simulink model "gtm_design_baseline3"  (R2023b)
settings: Solver=ode3  StartTime=0.0  StopTime=15  FixedStep=Timestep  MaxStep=.1  RelTol=1e-5
StopFcn:
  | MWSout=grabmws(bdroot);
  | MWSout.lastrun=datestr(now);
values from neighbouring files (symbols this model uses):
  f0_att = fc_att*Kb_att/Kb_rate    (= 0.125)    [runmain.m]    (also in runmain_match.m = 0.05)
  fc_att = 1/2    (= 0.5)    [runmain.m]    (also in runmain_match.m)
  fc_rate = 1/2    (= 0.5)    [runmain.m]    (also in runmain_match.m = 0)
  fi_att = 1/4    (= 0.25)    [runmain.m]    (also in runmain_match.m)
  fi_rate = 1/4    (= 0.25)    [runmain.m]    (also in runmain_match.m)
  flag_cmd = 0    [runmain.m]    (also in runmain_match.m)
  invBmat = inv(Bmat)    [runmain.m]    (also in runmain_match.m)
  invJ = inv(J)    [runmain.m]    (also in runmain_match.m)
  J = [Ixx 0 -Ixz; 0 Iyy 0; -Ixz 0 Izz]    [runmain.m]    (also in runmain_match.m)
  Kb_att = 1    [runmain.m]    (also in runmain_match.m)
  Kb_rate = 4    [runmain.m]    (also in runmain_match.m = 10)
  mws_designpoint = trimgtm(struct('eas',75,'gamma',0),'elev',1)    [runmain.m]    (also in runmain_match.m = trimgtm(struct('eas',90,'gamma',0),'elev',1))
undefined symbols (not defined in the file or in its folder): Aero, aftfuel, aftfuel_pos, b, bias, Cbar, cg_pos0, cg_shift_gear, DamageCase, DamageModels, DamageOnsetTime, engl_ang, engl_pos, engr_ang, engr_pos, fwdfuel, fwdfuel_pos, Inertia0, Inertia_shift_gear, ref_cg, runway_alt, S, StatesInp, symmetric_aero_on, Timestep, w0, WindDir, WindSpd
libraries: simulink_need_slupdate x56, Servo_Model_lib x18, Cross_Product_3D_lib x5, simulink x5, GTM_aerolib x4, Polyval_lib x3, Euler_to_DCM_lib x2, eomlib x2, Vb_Converter_lib x1, sensors_T2_design_lib x1, Doublet_Generator_lib x1, NamedStore_lib x1
(part 2 of 4)

== system gtm_design_baseline3/Aircraft Model/EOM/State Labels ==
  I : Inport
  Bus Creator : BusCreator  Inputs=12
  Demux : Demux  Outputs=12
      settings: DisplayOption=none
  O : Outport  VectorParamsAs1DForOutWhenUnconnected=off
  wires:
  Demux/12 -> Bus Creator/12  "psi"
  Demux/9 -> Bus Creator/9  "altitude"
  Demux/8 -> Bus Creator/8  "longitude"
  Demux/7 -> Bus Creator/7  "latitude"
  Demux/6 -> Bus Creator/6  "rb"
  Demux/5 -> Bus Creator/5  "qb"
  Demux/4 -> Bus Creator/4  "pb"
  Demux/3 -> Bus Creator/3  "wb"
  Demux/2 -> Bus Creator/2  "vb"
  Demux/1 -> Bus Creator/1  "ub"
  I/1 -> Demux/1
  Demux/10 -> Bus Creator/10  "phi"
  Demux/11 -> Bus Creator/11  "theta"
  Bus Creator/1 -> O/1

== system gtm_design_baseline3/Aircraft Model/EOM/Xdot Labels ==
  I : Inport
  Bus Creator : BusCreator  Inputs=12
  Demux : Demux  Outputs=12
      settings: DisplayOption=none
  O : Outport  VectorParamsAs1DForOutWhenUnconnected=off
  wires:
  Bus Creator/1 -> O/1
  Demux/11 -> Bus Creator/11  "theta_dot"
  Demux/10 -> Bus Creator/10  "phi_dot"
  I/1 -> Demux/1
  Demux/1 -> Bus Creator/1  "ub_dot"
  Demux/2 -> Bus Creator/2  "vb_dot"
  Demux/3 -> Bus Creator/3  "wb_dot"
  Demux/4 -> Bus Creator/4  "pb_dot"
  Demux/5 -> Bus Creator/5  "qb_dot"
  Demux/6 -> Bus Creator/6  "rb_dot"
  Demux/7 -> Bus Creator/7  "latitude_dot"
  Demux/8 -> Bus Creator/8  "longitude_dot"
  Demux/9 -> Bus Creator/9  "altitude_dot"
  Demux/12 -> Bus Creator/12  "psi_dot"

== system gtm_design_baseline3/Aircraft Model/Engines/3D Vector Cross Product ==
  A : Inport
  B : Inport  Port=2
  Demux : Demux  Outputs=3
      settings: DisplayOption=none
  Demux1 : Demux  Outputs=3
      settings: DisplayOption=none
  Gain : Gain  Gain=-1  SaturateOnIntegerOverflow=on  OutDataTypeStr=Inherit: Same as input  ParamDataTypeStr=Inherit: Same as input
  Ground : Ground
  Mux : Mux  Inputs=9
  Product : Product  Multiplication=Matrix(*)  SaturateOnIntegerOverflow=on  OutDataTypeStr=Inherit: Same as first input
  Reshape : Reshape  OutputDimensionality=Customize  OutputDimensions=[3,3]
  AxB : Outport  VectorParamsAs1DForOutWhenUnconnected=off
  wires:
  B/1 -> Product/2
  Reshape/1 -> Product/1
  Mux/1 -> Reshape/1
  Demux1/1 -> Mux/8
  Demux/2 -> Mux/7
  Demux/1 -> Mux/6
  Demux1/3 -> Mux/4
  Demux1/2 -> Mux/3
  Demux/3 -> Mux/2
  Gain/1 -> Demux1/1
  Ground/1 -> Mux/9, Mux/5, Mux/1
  Product/1 -> AxB/1
  A/1 -> Gain/1, Demux/1

== system gtm_design_baseline3/Aircraft Model/Engines/CG torque ==
  AC : Inport
  Lthrust : Inport  Port=2
  Rthrust : Inport  Port=3
  3D Vector Cross Product : Cross_Product_3D_lib/3D Vector Cross Product  SystemSampleTime=-1  VariantActivationTime=update diagram  AllowFlexibleInterface=on  Latency=0  AutoFrameSizeCalculation=off
  3D Vector Cross Product1 : Cross_Product_3D_lib/3D Vector Cross Product  SystemSampleTime=-1  VariantActivationTime=update diagram  AllowFlexibleInterface=on  Latency=0  AutoFrameSizeCalculation=off
  Bus Selector30 : BusSelector  OutputSignals=LfEng,CG,RtEng
  Sum1 : Sum  InputSameDT=on  SaturateOnIntegerOverflow=on  OutDataTypeStr=Inherit: Same as first input
  Sum6 : Sum  Inputs=+-  InputSameDT=on  SaturateOnIntegerOverflow=on  OutDataTypeStr=Inherit: Same as first input
  Sum7 : Sum  Inputs=-+  InputSameDT=on  SaturateOnIntegerOverflow=on  OutDataTypeStr=Inherit: Same as first input
  Torques : Outport  VectorParamsAs1DForOutWhenUnconnected=off
  wires:
  AC/1 -> Bus Selector30/1
  Bus Selector30/2 -> Sum7/1, Sum6/2  "<CG>"
  Lthrust/1 -> 3D Vector Cross Product1/2
  Rthrust/1 -> 3D Vector Cross Product/2
  Sum7/1 -> 3D Vector Cross Product/1
  Sum6/1 -> 3D Vector Cross Product1/1
  3D Vector Cross Product1/1 -> Sum1/1
  3D Vector Cross Product/1 -> Sum1/2
  Sum1/1 -> Torques/1
  Bus Selector30/3 -> Sum7/2  "<RtEng>"
  Bus Selector30/1 -> Sum6/1  "<LfEng>"

== system gtm_design_baseline3/Aircraft Model/Engines/Jetcat P70 (Left) ==
  note: No longer "halved"
  Throttle : Inport
  pratio : Inport  Port=2
  tratio : Inport  Port=3
  BypassDynamics : Inport  Port=4
  Fuel Pump Voltage : Lookup  InputValues=fuelflow_table  Table=fuelpump_table  LookUpMeth=Interpolation-Use End Values  SaturateOnIntegerOverflow=off
  Product2 : Product  RndMeth=Zero
  RPMref_2_EGT : Polyval  Coefs=Coeff_EGT
  RPMref_2_FuelFlow : Polyval  Coefs=Coeff_fuelflow
  RPMref_2_Thrust : Polyval  Coefs=Coeff_thrust
  Sum : Sum  Inputs=|+-
  Switch : Switch  Criteria=u2 ~= 0  SaturateOnIntegerOverflow=off  InputSameDT=off
  Terminator : Terminator
  Throttle1 : InportShadow
  Throttle2 : InportShadow
  Throttle_2_RPMref : Polyval  Coefs=Coeff_throttle
  Tunable Lag : Subsystem
  UnScale_Ref_RPM : Gain  Gain=123000/100
  Variable Lag : MATLAB Function  TreatAsAtomicUnit=on
  angular momentum : Gain  Gain=(pi*shaft_dia^4/32) * shaft_len * density * (2*pi/60)
  Thrust (lbf) : Outport  VectorParamsAs1DForOutWhenUnconnected=off
  RPM : Outport  Port=2  VectorParamsAs1DForOutWhenUnconnected=off
  h (slg-ft^2/s) : Outport  Port=3  VectorParamsAs1DForOutWhenUnconnected=off
  Fuel Flow (lbs/min) : Outport  Port=4  VectorParamsAs1DForOutWhenUnconnected=off
  Fuel Pump Voltage (V) : Outport  Port=5  VectorParamsAs1DForOutWhenUnconnected=off
  EGT (deg C) : Outport  Port=6  VectorParamsAs1DForOutWhenUnconnected=off
  wires:
  Throttle2/1 -> Switch/1
  BypassDynamics/1 -> Switch/2
  Tunable Lag/1(y) -> Switch/3, Sum/2  "Throttle_Lag"
  Switch/1 -> Throttle_2_RPMref/1
  Variable Lag/1(tau) -> Tunable Lag/1(tau)  "tau"
  Throttle/1 -> Tunable Lag/2(throttle)
  Throttle_2_RPMref/1 -> RPMref_2_EGT/1, Variable Lag/1(pa), RPMref_2_Thrust/1, UnScale_Ref_RPM/1, RPMref_2_FuelFlow/1
  angular momentum/1 -> h (slg-ft^2/s)/1
  UnScale_Ref_RPM/1 -> angular momentum/1, RPM/1
  tratio/1 -> Terminator/1
  RPMref_2_Thrust/1 -> Product2/1
  Product2/1 -> Thrust (lbf)/1
  RPMref_2_FuelFlow/1 -> Fuel Flow (lbs/min)/1, Fuel Pump Voltage/1
  pratio/1 -> Product2/2
  Fuel Pump Voltage/1 -> Fuel Pump Voltage (V)/1
  RPMref_2_EGT/1 -> EGT (deg C)/1
  Sum/1 -> Variable Lag/2(dp)
  Throttle1/1 -> Sum/1

== system gtm_design_baseline3/Aircraft Model/Engines/Jetcat P70 (Right) ==
  note: No longer "halved"
  Throttle : Inport
  pratio : Inport  Port=2
  tratio : Inport  Port=3
  BypassDynamics : Inport  Port=4
  Fuel Pump Voltage : Lookup  InputValues=fuelflow_table  Table=fuelpump_table  LookUpMeth=Interpolation-Use End Values  SaturateOnIntegerOverflow=off
  Product2 : Product  RndMeth=Zero
  RPMref_2_EGT : Polyval  Coefs=Coeff_EGT
  RPMref_2_FuelFlow : Polyval  Coefs=Coeff_fuelflow
  RPMref_2_Thrust : Polyval  Coefs=Coeff_thrust
  Sum : Sum  Inputs=|+-
  Switch : Switch  Criteria=u2 ~= 0  SaturateOnIntegerOverflow=off  InputSameDT=off
  Terminator : Terminator
  Throttle1 : InportShadow
  Throttle2 : InportShadow
  Throttle_2_RPMref : Polyval  Coefs=Coeff_throttle
  Tunable Lag : Subsystem
  UnScale_Ref_RPM : Gain  Gain=123000/100
  Variable Lag : MATLAB Function  TreatAsAtomicUnit=on
  angular momentum : Gain  Gain=(pi*shaft_dia^4/32) * shaft_len * density * (2*pi/60)
  Thrust (lbf) : Outport  VectorParamsAs1DForOutWhenUnconnected=off
  RPM : Outport  Port=2  VectorParamsAs1DForOutWhenUnconnected=off
  h (slg-ft^2/s) : Outport  Port=3  VectorParamsAs1DForOutWhenUnconnected=off
  Fuel Flow (lbs/min) : Outport  Port=4  VectorParamsAs1DForOutWhenUnconnected=off
  Fuel Pump Voltage (V) : Outport  Port=5  VectorParamsAs1DForOutWhenUnconnected=off
  EGT (deg C) : Outport  Port=6  VectorParamsAs1DForOutWhenUnconnected=off
  wires:
  Throttle2/1 -> Switch/1
  BypassDynamics/1 -> Switch/2
  Tunable Lag/1(y) -> Switch/3, Sum/2  "Throttle_Lag"
  Switch/1 -> Throttle_2_RPMref/1
  Variable Lag/1(tau) -> Tunable Lag/1(tau)  "tau"
  Throttle/1 -> Tunable Lag/2(throttle)
  Throttle_2_RPMref/1 -> RPMref_2_FuelFlow/1, RPMref_2_EGT/1, RPMref_2_Thrust/1, UnScale_Ref_RPM/1, Variable Lag/1(pa)
  angular momentum/1 -> h (slg-ft^2/s)/1
  UnScale_Ref_RPM/1 -> angular momentum/1, RPM/1
  tratio/1 -> Terminator/1
  RPMref_2_Thrust/1 -> Product2/1
  Product2/1 -> Thrust (lbf)/1
  RPMref_2_FuelFlow/1 -> Fuel Flow (lbs/min)/1, Fuel Pump Voltage/1
  pratio/1 -> Product2/2
  Fuel Pump Voltage/1 -> Fuel Pump Voltage (V)/1
  RPMref_2_EGT/1 -> EGT (deg C)/1
  Sum/1 -> Variable Lag/2(dp)
  Throttle1/1 -> Sum/1

== system gtm_design_baseline3/Aircraft Model/LandingGear/LandingForces ==
  h : Inport
  Xeom : Inport  Port=2
  Cmd : Inport  Port=3
  Enable : EnablePort
  Bus Selector1 : BusSelector  OutputSignals=STEER
  Bus Selector3 : BusSelector  OutputSignals=BRAKE
  Bus to Vector6 : BusToVector
  Embedded MATLAB Function : MATLAB Function  TreatAsAtomicUnit=on
  Gain : Gain  Gain=-1*NoseWheelRate
  Saturation +/-0.5 : Saturate
  Forces : Outport  InitialOutput=zeros(6,1)  VectorParamsAs1DForOutWhenUnconnected=off
  wires:
  Bus to Vector6/1 -> Embedded MATLAB Function/4(Xeom)
  Saturation +/-0.5/1 -> Embedded MATLAB Function/3(steerc)
  Gain/1 -> Saturation +/-0.5/1
  h/1 -> Embedded MATLAB Function/1(h)
  Xeom/1 -> Bus to Vector6/1
  Embedded MATLAB Function/1(F) -> Forces/1
  Cmd/1 -> Bus Selector3/1, Bus Selector1/1
  Bus Selector1/1 -> Gain/1  "<STEER>"
  Bus Selector3/1 -> Embedded MATLAB Function/2(brakec)  "<BRAKE>"

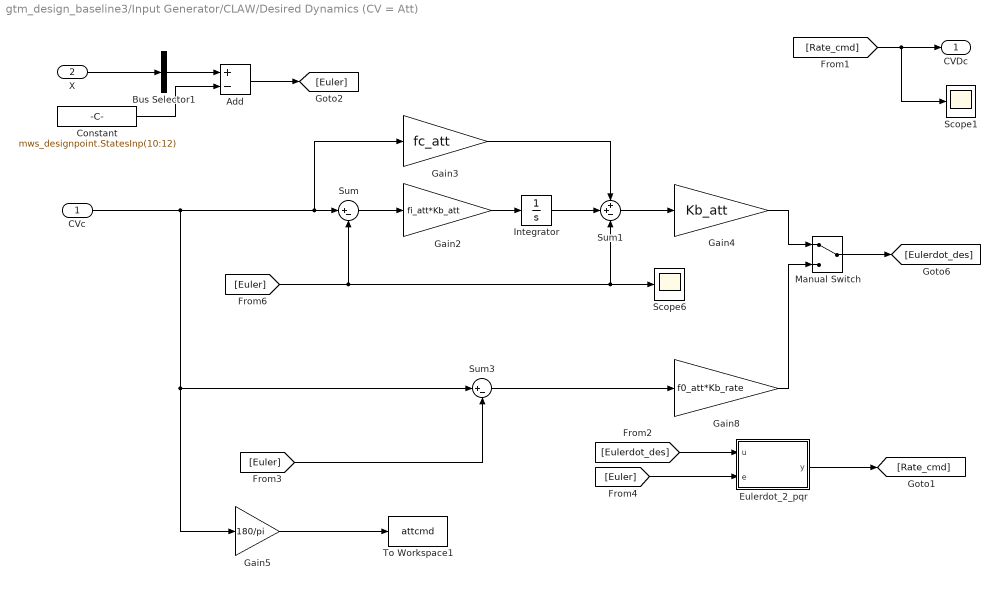
== system gtm_design_baseline3/Input Generator/CLAW/Desired Dynamics (CV = Att) ==
  CVc : Inport
  X : Inport  Port=2
  Add : Sum  Inputs=+-
  Bus Selector1 : BusSelector  OutputSignals=phi,theta,psi  OutputAsBus=on
  Constant : Constant  Value=mws_designpoint.StatesInp(10:12)
  Eulerdot_2_pqr : MATLAB Function  TreatAsAtomicUnit=on
  Gain2 : Gain  Gain=fi_att*Kb_att  SaturateOnIntegerOverflow=on  OutDataTypeStr=Inherit: Same as input  ParamDataTypeStr=Inherit: Same as input
  Gain3 : Gain  Gain=fc_att  SaturateOnIntegerOverflow=on  OutDataTypeStr=Inherit: Same as input  ParamDataTypeStr=Inherit: Same as input
  Gain4 : Gain  Gain=Kb_att  SaturateOnIntegerOverflow=on  OutDataTypeStr=Inherit: Same as input  ParamDataTypeStr=Inherit: Same as input
  Gain5 : Gain  Gain=180/pi  SaturateOnIntegerOverflow=on  OutDataTypeStr=Inherit: Same as input  ParamDataTypeStr=Inherit: Same as input
  Gain8 : Gain  Gain=f0_att*Kb_rate  SaturateOnIntegerOverflow=on  OutDataTypeStr=Inherit: Same as input  ParamDataTypeStr=Inherit: Same as input
  Integrator : Integrator
  Manual Switch : ManualSwitch
  Scope1 : Scope
  Scope6 : Scope
  Sum : Sum  Inputs=|+-
  Sum1 : Sum  Inputs=++-
  Sum3 : Sum  Inputs=|+-
  To Workspace1 : ToWorkspace  VariableName=attcmd  SaveFormat=Structure With Time  SampleTime=-1
  CVDc : Outport
  wires:
  [Rate_cmd] -> CVDc/1, Scope1/1
  X/1 -> Bus Selector1/1
  Sum1/1 -> Gain4/1
  Integrator/1 -> Sum1/2
  Gain3/1 -> Sum1/1
  Gain2/1 -> Integrator/1
  Sum/1 -> Gain2/1
  [Euler] -> Scope6/1, Sum1/3, Sum/2
  [Eulerdot_des] -> Eulerdot_2_pqr/1(u)
  CVc/1 -> Gain3/1, Sum/1, Gain5/1, Sum3/1
  Bus Selector1/1 -> Add/1
  Add/1 -> [Euler]
  Constant/1 -> Add/2
  Sum3/1 -> Gain8/1
  [Euler] -> Sum3/2
  Gain5/1 -> To Workspace1/1
  Eulerdot_2_pqr/1(y) -> [Rate_cmd]
  [Euler] -> Eulerdot_2_pqr/2(e)
  Gain4/1 -> Manual Switch/1
  Gain8/1 -> Manual Switch/2
  Manual Switch/1 -> [Eulerdot_des]

== system gtm_design_baseline3/Input Generator/CLAW/Desired Dynamics (CV = Rate) ==
  CVc : Inport
  X : Inport  Port=2
  Bus Selector1 : BusSelector  OutputSignals=pb,qb,rb  OutputAsBus=on
  Gain2 : Gain  Gain=fi_rate*Kb_rate  SaturateOnIntegerOverflow=on  OutDataTypeStr=Inherit: Same as input  ParamDataTypeStr=Inherit: Same as input
  Gain3 : Gain  Gain=fc_rate  SaturateOnIntegerOverflow=on  OutDataTypeStr=Inherit: Same as input  ParamDataTypeStr=Inherit: Same as input
  Gain4 : Gain  Gain=Kb_rate  SaturateOnIntegerOverflow=on  OutDataTypeStr=Inherit: Same as input  ParamDataTypeStr=Inherit: Same as input
  Gain5 : Gain  Gain=180/pi  SaturateOnIntegerOverflow=on  OutDataTypeStr=Inherit: Same as input  ParamDataTypeStr=Inherit: Same as input
  Integrator : Integrator
  Scope4 : Scope
  Scope6 : Scope
  Sum : Sum  Inputs=|+-
  Sum1 : Sum  Inputs=++-
  To Workspace : ToWorkspace  VariableName=ratecmd  SaveFormat=Structure With Time  SampleTime=-1
  CVDdes : Outport
  wires:
  CVc/1 -> Sum/1, Gain3/1, Scope4/1, Gain5/1
  [Omega] -> Sum/2, Sum1/3, Scope6/1
  Sum/1 -> Gain2/1
  Gain2/1 -> Integrator/1
  Gain3/1 -> Sum1/1
  Integrator/1 -> Sum1/2
  Sum1/1 -> Gain4/1
  Gain4/1 -> [Omegadot_des]
  X/1 -> Bus Selector1/1
  Bus Selector1/1 -> [Omega]
  [Omegadot_des] -> CVDdes/1
  Gain5/1 -> To Workspace/1

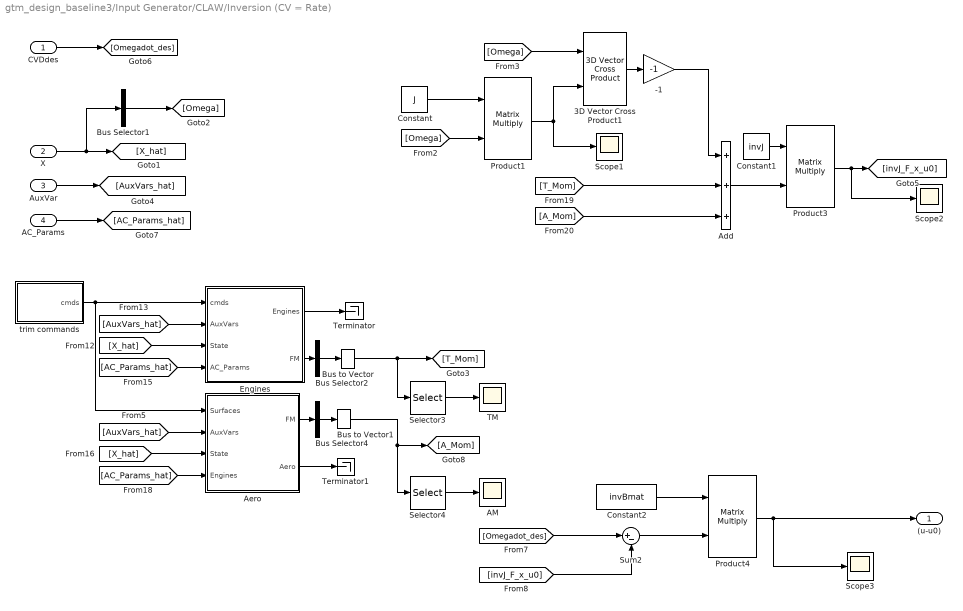
== system gtm_design_baseline3/Input Generator/CLAW/Inversion (CV = Rate) ==
  CVDdes : Inport
  X : Inport  Port=2
  AuxVar : Inport  Port=3
  AC_Params : Inport  Port=4
  -1 : Gain  Gain=-1  SaturateOnIntegerOverflow=on  OutDataTypeStr=Inherit: Same as input  ParamDataTypeStr=Inherit: Same as input
  3D Vector Cross Product1 : Cross_Product_3D_lib/3D Vector Cross Product  SystemSampleTime=-1  VariantActivationTime=update diagram  AllowFlexibleInterface=on  Latency=0  AutoFrameSizeCalculation=off
  AM : Scope
  Add : Sum  Inputs=+++
  Aero : Subsystem
  Bus Selector1 : BusSelector  OutputSignals=pb,qb,rb  OutputAsBus=on
  Bus Selector2 : BusSelector  OutputSignals=TLB,TMB,TNB  OutputAsBus=on
  Bus Selector4 : BusSelector  OutputSignals=LB,MB,NB  OutputAsBus=on
  Bus to Vector : BusToVector
  Bus to Vector1 : BusToVector
  Constant : Constant  Value=J
  Constant1 : Constant  Value=invJ
  Constant2 : Constant  Value=invBmat
  Engines : Subsystem
  Product1 : Product  Multiplication=Matrix(*)  RndMeth=Zero
  Product3 : Product  Multiplication=Matrix(*)  RndMeth=Zero
  Product4 : Product  Multiplication=Matrix(*)  RndMeth=Zero
  Scope1 : Scope
  Scope2 : Scope
  Scope3 : Scope
  Selector3 : Selector  InputPortWidth=3  IndexOptions=Index vector (dialog)  Indices=2  OutputSizes=1
  Selector4 : Selector  InputPortWidth=3  IndexOptions=Index vector (dialog)  Indices=2  OutputSizes=1
  Sum2 : Sum  Inputs=|+-
  TM : Scope
  Terminator : Terminator
  Terminator1 : Terminator
  trim commands : Subsystem
  (u-u0) : Outport
  wires:
  Constant/1 -> Product1/1
  [Omega] -> Product1/2
  [Omega] -> 3D Vector Cross Product1/1
  Product1/1 -> 3D Vector Cross Product1/2, Scope1/1
  3D Vector Cross Product1/1 -> -1/1
  -1/1 -> Add/1
  Add/1 -> Product3/2
  Constant1/1 -> Product3/1
  Product3/1 -> [invJ_F_x_u0], Scope2/1
  [T_Mom] -> Add/2
  [Omegadot_des] -> Sum2/1
  Constant2/1 -> Product4/1
  Sum2/1 -> Product4/2
  Product4/1 -> Scope3/1, (u-u0)/1
  [invJ_F_x_u0] -> Sum2/2
  [A_Mom] -> Add/3
  [X_hat] -> Engines/3(State)
  [AuxVars_hat] -> Engines/2(AuxVars)
  [AC_Params_hat] -> Engines/4(AC_Params)
  trim commands/1(cmds) -> Aero/1(Surfaces), Engines/1(cmds)
  Engines/2(FM) -> Bus Selector2/1
  Bus Selector2/1 -> Bus to Vector/1
  Bus to Vector/1 -> [T_Mom], Selector3/1
  [AuxVars_hat] -> Aero/2(AuxVars)
  [X_hat] -> Aero/3(State)
  [AC_Params_hat] -> Aero/4(Engines)
  Bus Selector4/1 -> Bus to Vector1/1
  Bus to Vector1/1 -> [A_Mom], Selector4/1
  Aero/1(FM) -> Bus Selector4/1
  Selector3/1 -> TM/1
  Selector4/1 -> AM/1
  X/1 -> [X_hat], Bus Selector1/1
  AuxVar/1 -> [AuxVars_hat]
  AC_Params/1 -> [AC_Params_hat]
  Bus Selector1/1 -> [Omega]
  CVDdes/1 -> [Omegadot_des]
  Engines/1(Engines) -> Terminator/1
  Aero/2(Aero) -> Terminator1/1

== system gtm_design_baseline3/Input Generator/CLAW/State Labels ==
  I : Inport
  Bus Creator : BusCreator  Inputs=12
  Demux : Demux  Outputs=12
      settings: DisplayOption=none
  O : Outport  VectorParamsAs1DForOutWhenUnconnected=off
  wires:
  Demux/12 -> Bus Creator/12  "psi"
  Demux/9 -> Bus Creator/9  "altitude"
  Demux/8 -> Bus Creator/8  "longitude"
  Demux/7 -> Bus Creator/7  "latitude"
  Demux/6 -> Bus Creator/6  "rb"
  Demux/5 -> Bus Creator/5  "qb"
  Demux/4 -> Bus Creator/4  "pb"
  Demux/3 -> Bus Creator/3  "wb"
  Demux/2 -> Bus Creator/2  "vb"
  Demux/1 -> Bus Creator/1  "ub"
  I/1 -> Demux/1
  Demux/10 -> Bus Creator/10  "phi"
  Demux/11 -> Bus Creator/11  "theta"
  Bus Creator/1 -> O/1

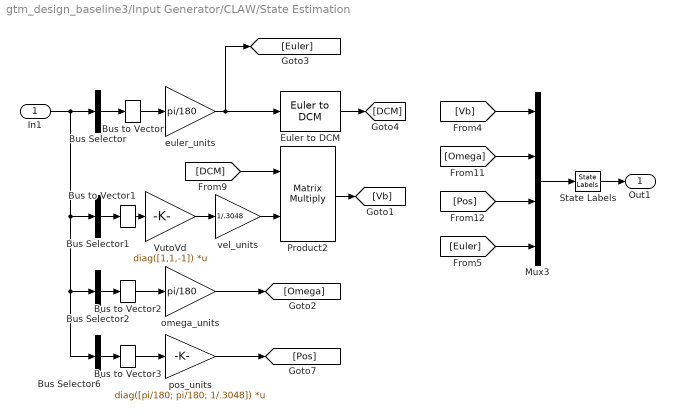
== system gtm_design_baseline3/Input Generator/CLAW/State Estimation ==
  In1 : Inport
  Bus Selector : BusSelector  OutputSignals=MIDG.phi_deg,MIDG.theta_deg,MIDG.psi_deg  OutputAsBus=on
  Bus Selector1 : BusSelector  OutputSignals=MIDG.NAV_Vn_mps,MIDG.NAV_Ve_mps,MIDG.NAV_Vu_mps  OutputAsBus=on
  Bus Selector2 : BusSelector  OutputSignals=MAG3.p_deg,MAG3.q_deg,MAG3.r_deg  OutputAsBus=on
  Bus Selector6 : BusSelector  OutputSignals=MIDG.NAV_latitude_deg,MIDG.NAV_longitude_deg,MIDG.NAV_altitude_m  OutputAsBus=on
  Bus to Vector{,1..3} (4 alike) : BusToVector
  Euler to DCM : Euler_to_DCM_lib/Euler to DCM  SystemSampleTime=-1  VariantActivationTime=update diagram  AllowFlexibleInterface=on  Latency=0  AutoFrameSizeCalculation=off
  Mux3 : Mux  Inputs=[3 3 3 3]
  Product2 : Product  Multiplication=Matrix(*)  RndMeth=Zero
  State Labels : eomlib/EOM/State Labels  SystemSampleTime=-1  VariantActivationTime=update diagram  AllowFlexibleInterface=on  Latency=0  AutoFrameSizeCalculation=off
  VutoVd : Gain  Gain=diag([1,1,-1])  Multiplication=Matrix(K*u)  SaturateOnIntegerOverflow=on  OutDataTypeStr=Inherit: Same as input  ParamDataTypeStr=Inherit: Same as input
  euler_units : Gain  Gain=pi/180  SaturateOnIntegerOverflow=on  OutDataTypeStr=Inherit: Same as input  ParamDataTypeStr=Inherit: Same as input
  omega_units : Gain  Gain=pi/180  SaturateOnIntegerOverflow=on  OutDataTypeStr=Inherit: Same as input  ParamDataTypeStr=Inherit: Same as input
  pos_units : Gain  Gain=diag([pi/180; pi/180; 1/.3048])  Multiplication=Matrix(K*u)
  vel_units : Gain  Gain=1/.3048
  Out1 : Outport
  wires:
  In1/1 -> Bus Selector/1, Bus Selector1/1, Bus Selector2/1, Bus Selector6/1
  Bus Selector/1 -> Bus to Vector/1
  euler_units/1 -> [Euler], Euler to DCM/1
  Euler to DCM/1 -> [DCM]
  Bus Selector1/1 -> Bus to Vector1/1
  VutoVd/1 -> vel_units/1
  [DCM] -> Product2/1
  Product2/1 -> [Vb]
  Bus Selector2/1 -> Bus to Vector2/1
  omega_units/1 -> [Omega]
  Bus to Vector/1 -> euler_units/1
  Bus to Vector1/1 -> VutoVd/1
  Bus to Vector2/1 -> omega_units/1
  Bus Selector6/1 -> Bus to Vector3/1
  pos_units/1 -> [Pos]
  Bus to Vector3/1 -> pos_units/1
  vel_units/1 -> Product2/2
  [Vb] -> Mux3/1
  [Omega] -> Mux3/2
  [Pos] -> Mux3/3
  [Euler] -> Mux3/4
  Mux3/1 -> State Labels/1
  State Labels/1 -> Out1/1

== system gtm_design_baseline3/Aircraft Model/A//C parameters/Inertia//Mass//CG Shift/DamageEffects ==
  In : Inport
  Gain1 : Constant  Value=dInertiaDamage
  Squeeze2 : Squeeze
  Value(ndx,:) : Selector  NumberOfDimensions=2  IndexMode=Zero-based  InputPortWidth=3  IndexOptions=Index vector (port),Select all  Indices=[1 3],1  OutputSizes=1,1
  dInertia : Outport  VectorParamsAs1DForOutWhenUnconnected=off
  wires:
  Squeeze2/1 -> dInertia/1
  Value(ndx,:)/1 -> Squeeze2/1
  Gain1/1 -> Value(ndx,:)/1
  In/1 -> Value(ndx,:)/2

== system gtm_design_baseline3/Aircraft Model/A//C parameters/Inertia//Mass//CG Shift/FuelBurnEffects ==
  In : Inport
  Mux : Mux
  Polyval : Polyval_lib/Polyval  p=Ixx_model
  Polyval1 : Polyval_lib/Polyval  p=Iyy_model
  Polyval2 : Polyval_lib/Polyval  p=Izz_model
  xCG6 : Constant  Value=zeros(1,3)
  dInertia : Outport  VectorParamsAs1DForOutWhenUnconnected=off
  wires:
  Mux/1 -> dInertia/1
  Polyval2/1 -> Mux/3
  Polyval1/1 -> Mux/2
  Polyval/1 -> Mux/1
  xCG6/1 -> Mux/4
  In/1 -> Polyval2/1, Polyval1/1, Polyval/1

== system gtm_design_baseline3/Aircraft Model/A//C parameters/Inertia//Mass//CG Shift/cg//weight ==
  DamageCase : Inport
  Gain1 : Constant  Value=dMassDamage
  Gain2 : Constant  Value=dCGDamage
  Squeeze1 : Squeeze
  Squeeze2 : Squeeze
  Value(ndx,:) : Selector  IndexMode=Zero-based  IndexOptions=Index vector (port)  Indices=[1 3]  OutputSizes=1
  Value(ndx,:)1 : Selector  NumberOfDimensions=2  IndexMode=Zero-based  InputPortWidth=3  IndexOptions=Index vector (port),Select all  Indices=[1 3],1  OutputSizes=1,1
  dCG : Outport  VectorParamsAs1DForOutWhenUnconnected=off
  dweight : Outport  Port=2  VectorParamsAs1DForOutWhenUnconnected=off
  wires:
  Squeeze2/1 -> dweight/1
  Squeeze1/1 -> dCG/1
  Value(ndx,:)/1 -> Squeeze2/1
  Gain1/1 -> Value(ndx,:)/1
  DamageCase/1 -> Value(ndx,:)1/2, Value(ndx,:)/2
  Value(ndx,:)1/1 -> Squeeze1/1
  Gain2/1 -> Value(ndx,:)1/1

== system gtm_design_baseline3/Aircraft Model/Aero/Coefficent Evaluation/3D Vector Cross Product ==
  A : Inport
  B : Inport  Port=2
  Demux : Demux  Outputs=3
      settings: DisplayOption=none
  Demux1 : Demux  Outputs=3
      settings: DisplayOption=none
  Gain : Gain  Gain=-1  SaturateOnIntegerOverflow=on  OutDataTypeStr=Inherit: Same as input  ParamDataTypeStr=Inherit: Same as input
  Ground : Ground
  Math Function : Math  Operator=transpose  SignedPower=on
  Mux : Mux  Inputs=9
  Product : Product  Multiplication=Matrix(*)  SaturateOnIntegerOverflow=on  OutDataTypeStr=Inherit: Same as first input
  Reshape : Reshape  OutputDimensionality=Customize  OutputDimensions=[3,3]
  AxB : Outport  VectorParamsAs1DForOutWhenUnconnected=off
  wires:
  A/1 -> Demux/1, Gain/1
  Product/1 -> AxB/1
  Ground/1 -> Mux/1, Mux/5, Mux/9
  Gain/1 -> Demux1/1
  Demux/3 -> Mux/2
  Demux1/2 -> Mux/3
  Demux1/3 -> Mux/4
  Demux/1 -> Mux/6
  Demux/2 -> Mux/7
  Demux1/1 -> Mux/8
  Mux/1 -> Reshape/1
  Reshape/1 -> Product/1
  B/1 -> Math Function/1
  Math Function/1 -> Product/2

== system gtm_design_baseline3/Aircraft Model/Aero/Dynamic Derviatives/Forced Oscillation with Damage Increments ==
  alpha : Inport
  TAS : Inport  Port=2
  pqr : Inport  Port=3
  AC_Params : Inport  Port=4
  DamageCase : Inport  Port=5
  Action Port : ActionPort  ActionPortLabel=case [ 1 2 3 4 5 6 ]:
  Add : Sum  Inputs=+++
  Add1 : Sum
  Assignment to CY : Assignment  IndexMode=Zero-based  IndexOptions=Index vector (dialog)  Indices=1  OutputSizes=[1 1]
  Constant4 : Constant  Value=zeros(6,1)
  Damage Effects-Increments : Subsystem
  Damage Effects-Scaling : Subsystem
  Forced Oscillation : Subsystem
  Normalize : Subsystem
  Product1 : Product  RndMeth=Zero
  Product2 : Product  RndMeth=Zero
  Product3 : Product  RndMeth=Zero
  dC6 : Outport
  wires:
  Assignment to CY/1 -> Add1/1
  Add/1 -> Add1/2
  Product2/1 -> Add/1
  Product1/1 -> Add/2
  Product3/1 -> Add/3
  Forced Oscillation/3(dC6_r) -> Product3/2
  Forced Oscillation/2(dC6_q) -> Product1/2
  Forced Oscillation/1(dC6_p) -> Product2/2
  Normalize/1(pqrhat) -> Damage Effects-Increments/2(pqr), Forced Oscillation/2(pqr)
  AC_Params/1 -> Normalize/3(AC_Params)
  TAS/1 -> Normalize/2(TAS)
  pqr/1 -> Normalize/1(pqr)
  Add1/1 -> dC6/1
  Constant4/1 -> Assignment to CY/1
  Damage Effects-Increments/1(Increment) -> Assignment to CY/2
  Damage Effects-Scaling/3(Scaling_p) -> Product2/1
  Damage Effects-Scaling/2(Scaling_q) -> Product1/1
  Damage Effects-Scaling/1(Scaling_r) -> Product3/1
  DamageCase/1 -> Damage Effects-Increments/3(DamageCase), Damage Effects-Scaling/2(DamageCase)
  alpha/1 -> Damage Effects-Increments/1(alpha), Damage Effects-Scaling/1(alpha), Forced Oscillation/1(alpha)

== system gtm_design_baseline3/Aircraft Model/Aero/Dynamic Derviatives/Rotary Blended UnDamaged Case ==
  alpha : Inport
  beta : Inport  Port=2
  TAS : Inport  Port=3
  pqr : Inport  Port=4
  AC_Params : Inport  Port=5
  Action Port : ActionPort  ActionPortLabel=default:
  Add : Sum  Inputs=++++
  Blending Function : MATLAB Function  TreatAsAtomicUnit=on
  Bus Selector2 : BusSelector  OutputSignals=B,Cbar
  Forced Oscillation : Subsystem
  Rotary Balance : Subsystem
  Saturation : Saturate
  Saturation1 : Saturate  UpperLimit=10000  LowerLimit=1
  dC6 : Outport
  wires:
  Forced Oscillation/3(dC6_r) -> Add/4
  Forced Oscillation/2(dC6_q) -> Add/3
  Forced Oscillation/1(dC6_p) -> Add/2
  Rotary Balance/1(dC6) -> Add/1
  Add/1 -> dC6/1
  Bus Selector2/2 -> Blending Function/6(Cbar)  "<Cbar>"
  pqr/1 -> Blending Function/4(pqr)
  Saturation1/1 -> Blending Function/3(tas)
  Saturation/1 -> Rotary Balance/3(w)
  [alpha] -> Forced Oscillation/1(alpha)
  [beta] -> Rotary Balance/2(beta)
  [alpha] -> Rotary Balance/1(alpha)
  [beta] -> Blending Function/2(beta)
  beta/1 -> [beta]
  alpha/1 -> [alpha]
  [alpha] -> Blending Function/1(alpha)
  AC_Params/1 -> Bus Selector2/1
  TAS/1 -> Saturation1/1
  Bus Selector2/1 -> Blending Function/5(B)  "<B>"
  Blending Function/2(pqr_osc) -> Forced Oscillation/2(pqr)
  Blending Function/1(omega) -> Saturation/1

== system gtm_design_baseline3/Aircraft Model/AuxiliaryVariables/Atmos76/Atmos List ==
  I : Inport
  BusCreator : BusCreator  Inputs=7
  Demux2 : Demux  Outputs=[1 1 1 1 1 1]
      settings: DisplayOption=none
  Divide : Product  Inputs=*/
  Standard Temp. K : Constant  Value=288.15
  O : Outport  VectorParamsAs1DForOutWhenUnconnected=off
  wires:
  Divide/1 -> BusCreator/7  "tratio"
  Standard Temp. K/1 -> Divide/2
  BusCreator/1 -> O/1
  I/1 -> Demux2/1
  Demux2/1 -> BusCreator/1  "rho"
  Demux2/2 -> BusCreator/2  "pressure"
  Demux2/3 -> Divide/1, BusCreator/3  "temperature"
  Demux2/4 -> BusCreator/4  "cs"
  Demux2/5 -> BusCreator/5  "pratio"
  Demux2/6 -> BusCreator/6  "sqrsig"

== system gtm_design_baseline3/Aircraft Model/EOM/Anti Windup/Subsystem1 ==
  I : Inport
  Constant1 : Constant  Value=2*pi
  Constant2 : Constant  Value=2*pi
  Constant3 : Constant  Value=2*pi
  Math Function1 : Math  Operator=rem  SignedPower=on
  Sum : Sum  Inputs=|-+  SaturateOnIntegerOverflow=on
  Sum1 : Sum  Inputs=++|  SaturateOnIntegerOverflow=on
  Switch : Switch  Criteria=u2 > Threshold  Threshold=pi  InputSameDT=off
  Switch1 : Switch  InputSameDT=off
  Switch2 : Switch  Threshold=-pi  InputSameDT=off
  O : Outport  VectorParamsAs1DForOutWhenUnconnected=off
  wires:
  Switch1/1 -> O/1
  Switch/1 -> Switch1/1
  Switch2/1 -> Switch1/3
  Sum1/1 -> Switch2/3
  Constant3/1 -> Sum1/2
  Sum/1 -> Switch/1
  Constant2/1 -> Sum/1
  Math Function1/1 -> Switch1/2, Sum1/1, Switch2/2, Switch2/1, Switch/3, Sum/2, Switch/2
  I/1 -> Math Function1/1
  Constant1/1 -> Math Function1/2

== system gtm_design_baseline3/Aircraft Model/EOM/Anti Windup/Subsystem3 ==
  I : Inport
  Constant1 : Constant  Value=2*pi
  Constant2 : Constant  Value=2*pi
  Constant3 : Constant  Value=2*pi
  Math Function1 : Math  Operator=rem  SignedPower=on
  Sum : Sum  Inputs=|-+  SaturateOnIntegerOverflow=on
  Sum1 : Sum  Inputs=++|  SaturateOnIntegerOverflow=on
  Switch : Switch  Criteria=u2 > Threshold  Threshold=pi  InputSameDT=off
  Switch1 : Switch  InputSameDT=off
  Switch2 : Switch  Threshold=-pi  InputSameDT=off
  O : Outport  VectorParamsAs1DForOutWhenUnconnected=off
  wires:
  Switch1/1 -> O/1
  Switch/1 -> Switch1/1
  Switch2/1 -> Switch1/3
  Sum1/1 -> Switch2/3
  Constant3/1 -> Sum1/2
  Sum/1 -> Switch/1
  Constant2/1 -> Sum/1
  Math Function1/1 -> Switch1/2, Sum1/1, Switch2/2, Switch2/1, Switch/3, Sum/2, Switch/2
  I/1 -> Math Function1/1
  Constant1/1 -> Math Function1/2

== system gtm_design_baseline3/Aircraft Model/EOM/Anti Windup/Subsystem4 ==
  I : Inport
  Constant1 : Constant  Value=2*pi
  Math Function1 : Math  Operator=rem  SignedPower=on
  Math Function2 : Math  Operator=rem  SignedPower=on
  Sum2 : Sum  Inputs=|++  SaturateOnIntegerOverflow=on
  O : Outport  VectorParamsAs1DForOutWhenUnconnected=off
  wires:
  Constant1/1 -> Math Function1/2, Math Function2/2, Sum2/2
  I/1 -> Math Function1/1
  Sum2/1 -> Math Function2/1
  Math Function1/1 -> Sum2/1
  Math Function2/1 -> O/1

== system gtm_design_baseline3/Aircraft Model/Engines/Jetcat P70 (Left)/Tunable Lag ==
  tau : Inport
  throttle : Inport  Port=2
  Integrator : Integrator  InitialConditionSource=external
  Product : Product  Inputs=/*  RndMeth=Zero
  Sum : Sum  Inputs=|+-
  y : Outport  VectorParamsAs1DForOutWhenUnconnected=off
  wires:
  throttle/1 -> Integrator/2, Sum/1
  tau/1 -> Product/1
  Sum/1 -> Product/2
  Product/1 -> Integrator/1
  Integrator/1 -> y/1, Sum/2  "Throttle_Lag"

== system gtm_design_baseline3/Aircraft Model/Engines/Jetcat P70 (Right)/Tunable Lag ==
  tau : Inport
  throttle : Inport  Port=2
  Integrator : Integrator  InitialConditionSource=external
  Product : Product  Inputs=/*  RndMeth=Zero
  Sum : Sum  Inputs=|+-
  y : Outport  VectorParamsAs1DForOutWhenUnconnected=off
  wires:
  throttle/1 -> Integrator/2, Sum/1
  tau/1 -> Product/1
  Sum/1 -> Product/2
  Product/1 -> Integrator/1
  Integrator/1 -> y/1, Sum/2  "Throttle_Lag"

== system gtm_design_baseline3/Input Generator/CLAW/Inversion (CV = Rate)/Aero ==
  Surfaces : Inport
  AuxVars : Inport  Port=2
  State : Inport  Port=3
  Engines : Inport  Port=4
  Basic Airframe : GTM_aerolib/Basic Airframe  SystemSampleTime=-1  VariantActivationTime=update diagram  AllowFlexibleInterface=on  Latency=0  AutoFrameSizeCalculation=off
  Bus Selector1 : BusSelector  OutputSignals=CG,CP
  Bus Selector2 : BusSelector  OutputSignals=alpha,beta
  Bus Selector6 : BusSelector  OutputSignals=tas
  Bus Selector7 : BusSelector  OutputSignals=qbar
  Bus Selector8 : BusSelector  OutputSignals=pb,qb,rb  OutputAsBus=on
  Bus to Vector5 : BusToVector
  Coefficent Evaluation : Subsystem  mask{b=b, cbar=Cbar, Sref=S}
      mask prompts: b "Reference Span (b)"; cbar "Reference Chord (cbar)"; Sref "Reference Area (Sref)"
      mask help:
      | Calulates the Force and Moments due to aerodynamic loads from vector of body axes aerodynamic coefficients:
      |    C6body = [Cx Cy Cz Cl Cm Cn].
      | Also requires dynamic pressure, cg/cp locations and reference lengths/area.
  Control Surfaces : GTM_aerolib/Control Surfaces  SystemSampleTime=-1  VariantActivationTime=update diagram  AllowFlexibleInterface=on  Latency=0  AutoFrameSizeCalculation=off
  Dynamic Derviatives : Subsystem  AncestorBlock=GTM_aerolib/Dynamic Derviatives
  Label : Subsystem
  Sum8 : Sum  Inputs=+++  InputSameDT=on  SaturateOnIntegerOverflow=on  OutDataTypeStr=Inherit: Same as first input
  Terminator : Terminator
  symmetry_on : Constant  Value=symmetric_aero_on
  FM : Outport  VectorParamsAs1DForOutWhenUnconnected=off
  Aero : Outport  Port=2  VectorParamsAs1DForOutWhenUnconnected=off
  wires:
  [AC_Params] -> Dynamic Derviatives/5(AC_Params)
  Bus to Vector5/1 -> Dynamic Derviatives/4(pqr)
  Bus Selector6/1 -> Dynamic Derviatives/3(TAS)  "<tas>"
  [AC_Params] -> Control Surfaces/4
  [AC_Params] -> Basic Airframe/4
  Bus Selector8/1 -> Bus to Vector5/1  "pqr"
  Engines/1 -> Terminator/1
  Basic Airframe/1 -> Sum8/1
  Control Surfaces/1 -> Sum8/2
  Dynamic Derviatives/1(dC6) -> Sum8/3
  State/1 -> Bus Selector8/1
  Bus Selector2/2 -> Basic Airframe/2, Dynamic Derviatives/2(beta), Control Surfaces/2  "<beta>"
  Bus Selector2/1 -> Basic Airframe/1, Dynamic Derviatives/1(alpha), Control Surfaces/1  "<alpha>"
  AuxVars/1 -> Bus Selector2/1, Bus Selector6/1, Bus Selector7/1
  Label/1(O) -> FM/1
  Bus Selector7/1 -> Coefficent Evaluation/2(qbar)  "<qbar>"
  Sum8/1 -> Aero/1, Coefficent Evaluation/1(C6 Body)
  Coefficent Evaluation/1(Forces) -> Label/1(If)
  Coefficent Evaluation/2(Moments) -> Label/2(Im)
  Bus Selector1/1 -> Coefficent Evaluation/3(Cg)  "<CG>"
  [AC_Params] -> Bus Selector1/1
  Bus Selector1/2 -> Coefficent Evaluation/4(Cp)  "<CP>"
  symmetry_on/1 -> Basic Airframe/3
  Surfaces/1 -> Control Surfaces/3

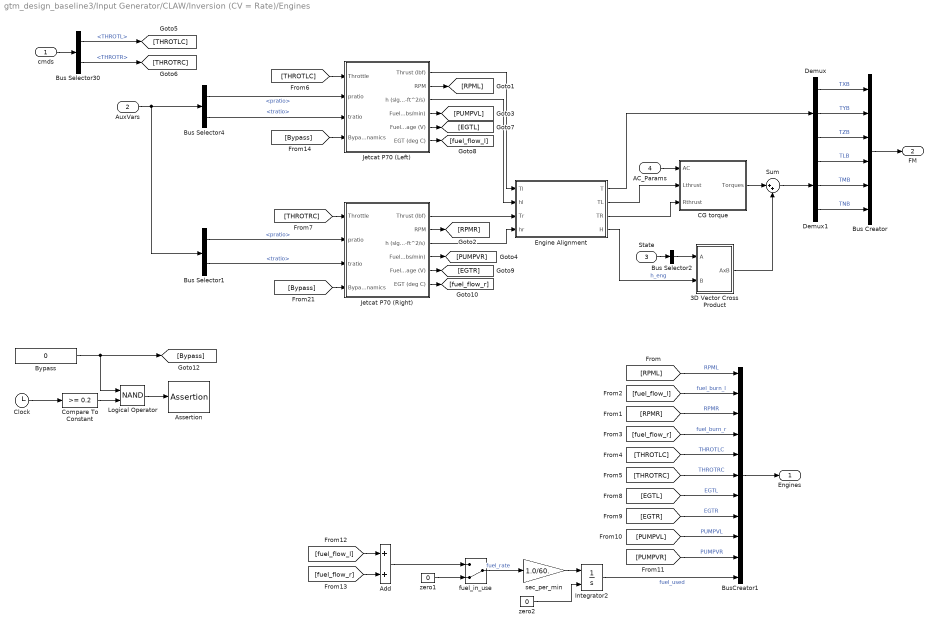
== system gtm_design_baseline3/Input Generator/CLAW/Inversion (CV = Rate)/Engines ==
  cmds : Inport
  AuxVars : Inport  Port=2
  State : Inport  Port=3
  AC_Params : Inport  Port=4
  3D Vector Cross Product : Subsystem
  Add : Sum
  Assertion : Assertion  AssertionFailFcn=warndlg('Engine dynamics in bypass mode. Run setup.m to reset.','Warning!')
  Bus Creator : BusCreator  Inputs=6
  Bus Selector1 : BusSelector  OutputSignals=pratio,tratio
  Bus Selector2 : BusSelector  OutputSignals=pb,qb,rb  OutputAsBus=on
  Bus Selector30 : BusSelector  OutputSignals=THROTL,THROTR
  Bus Selector4 : BusSelector  OutputSignals=pratio,tratio
  BusCreator1 : BusCreator  Inputs=11
  Bypass : Constant  Value=0
  CG torque : Subsystem
  Clock : Clock
  Compare To Constant : simulink/Logic and Bit Operations/Compare To Constant  relop=>=  const=0.2  OutDataTypeStr=boolean  ZeroCross=off
  Demux : Demux  Outputs=3
  Demux1 : Demux  Outputs=3
  Engine Alignment : MATLAB Function  TreatAsAtomicUnit=on
  Integrator2 : Integrator  InitialConditionSource=external
  Jetcat P70 (Left) : Subsystem
      mask init: same as gtm_design_baseline3/Aircraft Model/Engines/Jetcat P70 (Left)
  Jetcat P70 (Right) : Subsystem
      mask init: same as gtm_design_baseline3/Aircraft Model/Engines/Jetcat P70 (Left)
  Logical Operator : Logic  Operator=NAND  AllPortsSameDT=off  OutDataTypeStr=boolean
  Sum : Sum  Inputs=|++
  fuel_in_use : ManualSwitch  CurrentSetting=0
  sec_per_min : Gain  Gain=1.0/60.  SaturateOnIntegerOverflow=on  OutDataTypeStr=Inherit: Same as input  ParamDataTypeStr=Inherit: Same as input
  zero1 : Constant  Value=0
  zero2 : Constant  Value=0
  Engines : Outport  VectorParamsAs1DForOutWhenUnconnected=off
  FM : Outport  Port=2  PortDimensions=6  VectorParamsAs1DForOutWhenUnconnected=off
  wires:
  Jetcat P70 (Right)/6(EGT (deg C)) -> [fuel_flow_r]
  Jetcat P70 (Right)/5(Fuel Pump Voltage (V)) -> [EGTR]
  Jetcat P70 (Left)/6(EGT (deg C)) -> [fuel_flow_l]
  Jetcat P70 (Left)/5(Fuel Pump Voltage (V)) -> [EGTL]
  cmds/1 -> Bus Selector30/1
  Demux/2 -> Bus Creator/2  "TYB"
  State/1 -> Bus Selector2/1
  Bus Selector2/1 -> 3D Vector Cross Product/1(A)
  Demux/3 -> Bus Creator/3  "TZB"
  Jetcat P70 (Left)/2(RPM) -> [RPML]
  Jetcat P70 (Left)/4(Fuel Flow (lbs/min)) -> [PUMPVL]
  Jetcat P70 (Right)/4(Fuel Flow (lbs/min)) -> [PUMPVR]
  Jetcat P70 (Right)/2(RPM) -> [RPMR]
  Bus Selector1/1 -> Jetcat P70 (Right)/2(pratio)  "<pratio>"
  Bus Selector1/2 -> Jetcat P70 (Right)/3(tratio)  "<tratio>"
  AuxVars/1 -> Bus Selector1/1, Bus Selector4/1
  AC_Params/1 -> CG torque/1(AC)
  Bus Creator/1 -> FM/1
  Bus Selector30/1 -> [THROTLC]  "<THROTL>"
  Bus Selector30/2 -> [THROTRC]  "<THROTR>"
  [THROTLC] -> Jetcat P70 (Left)/1(Throttle)
  [THROTRC] -> Jetcat P70 (Right)/1(Throttle)
  [THROTRC] -> BusCreator1/6  "THROTRC"
  [THROTLC] -> BusCreator1/5  "THROTLC"
  [fuel_flow_r] -> BusCreator1/4  "fuel_burn_r"
  [fuel_flow_l] -> BusCreator1/2  "fuel_burn_l"
  [RPMR] -> BusCreator1/3  "RPMR"
  [RPML] -> BusCreator1/1  "RPML"
  BusCreator1/1 -> Engines/1
  [EGTL] -> BusCreator1/7  "EGTL"
  [EGTR] -> BusCreator1/8  "EGTR"
  [PUMPVL] -> BusCreator1/9  "PUMPVL"
  [PUMPVR] -> BusCreator1/10  "PUMPVR"
  sec_per_min/1 -> Integrator2/1
  fuel_in_use/1 -> sec_per_min/1  "fuel_rate"
  Integrator2/1 -> BusCreator1/11  "fuel_used"
  zero2/1 -> Integrator2/2
  [fuel_flow_l] -> Add/1
  [fuel_flow_r] -> Add/2
  zero1/1 -> fuel_in_use/2
  Add/1 -> fuel_in_use/1
  Bus Selector4/1 -> Jetcat P70 (Left)/2(pratio)  "<pratio>"
  Bus Selector4/2 -> Jetcat P70 (Left)/3(tratio)  "<tratio>"
  [Bypass] -> Jetcat P70 (Left)/4(BypassDynamics)
  [Bypass] -> Jetcat P70 (Right)/4(BypassDynamics)
  Bypass/1 -> Logical Operator/1, [Bypass]
  Clock/1 -> Compare To Constant/1
  Jetcat P70 (Left)/1(Thrust (lbf)) -> Engine Alignment/1(Tl)
  Jetcat P70 (Right)/1(Thrust (lbf)) -> Engine Alignment/3(Tr)
  Demux/1 -> Bus Creator/1  "TXB"
  Jetcat P70 (Left)/3(h (slg-ft^2/s)) -> Engine Alignment/2(hl)
  Jetcat P70 (Right)/3(h (slg-ft^2/s)) -> Engine Alignment/4(hr)
  Engine Alignment/4(H) -> 3D Vector Cross Product/2(B)  "h_eng"
  Engine Alignment/1(T) -> Demux/1
  Engine Alignment/2(TL) -> CG torque/2(Lthrust)
  Engine Alignment/3(TR) -> CG torque/3(Rthrust)
  CG torque/1(Torques) -> Sum/1
  3D Vector Cross Product/1(AxB) -> Sum/2
  Sum/1 -> Demux1/1
  Demux1/1 -> Bus Creator/4  "TLB"
  Demux1/2 -> Bus Creator/5  "TMB"
  Demux1/3 -> Bus Creator/6  "TNB"
  Compare To Constant/1 -> Logical Operator/2
  Logical Operator/1 -> Assertion/1

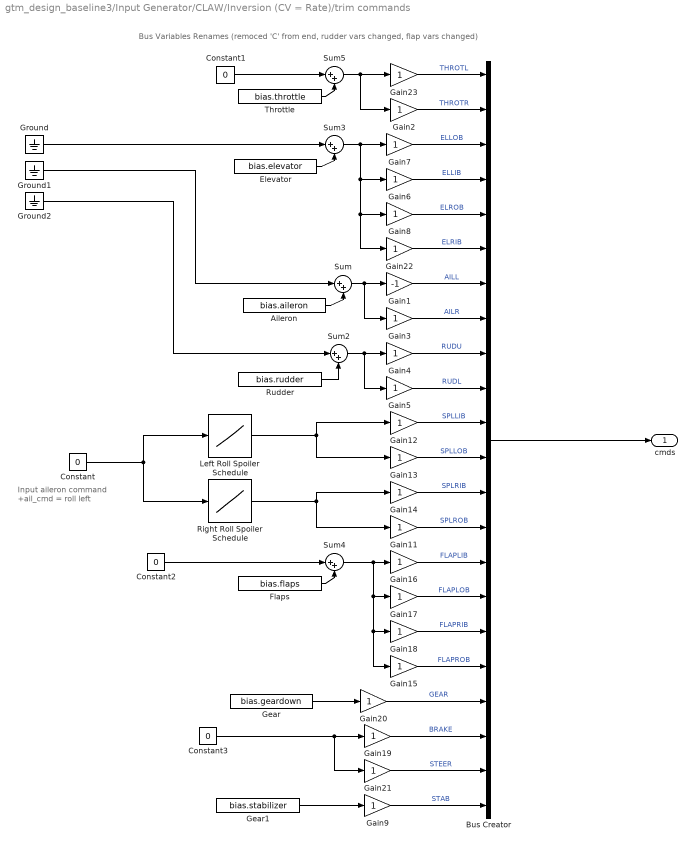
== system gtm_design_baseline3/Input Generator/CLAW/Inversion (CV = Rate)/trim commands ==
  note: Input aileron command
      | +ail_cmd = roll left
  note: Bus Variables Renames (remoced 'C' from end, rudder vars changed, flap vars changed)
  Aileron : Constant  Value=bias.aileron
  Bus Creator : BusCreator  Inputs=22
  Constant{,1..3} (4 alike) : Constant  Value=0
  Elevator : Constant  Value=bias.elevator
  Flaps : Constant  Value=bias.flaps
  Gain1 : Gain  Gain=-1  SaturateOnIntegerOverflow=on  OutDataTypeStr=Inherit: Same as input  ParamDataTypeStr=Inherit: Same as input
  Gain{2..9,11..23} (21 alike) : Gain  SaturateOnIntegerOverflow=on  OutDataTypeStr=Inherit: Same as input  ParamDataTypeStr=Inherit: Same as input
  Gear : Constant  Value=bias.geardown
  Gear1 : Constant  Value=bias.stabilizer
  Ground : Ground
  Ground1 : Ground
  Ground2 : Ground
  Left Roll Spoiler Schedule : Lookup  InputValues="[-20\t-11.76\t-2.36\t0\t2.36\t11.76\t20\t]"  Table=[0 0 0 0 0 9 45]  LookUpMeth=Interpolation-Use End Values  SaturateOnIntegerOverflow=off
  Right Roll Spoiler Schedule : Lookup  InputValues="[-20\t-11.76\t-2.36\t0\t2.36\t11.76\t20\t]"  Table=[45 9 0 0 0 0 0]  LookUpMeth=Interpolation-Use End Values  SaturateOnIntegerOverflow=off
  Rudder : Constant  Value=bias.rudder
  Sum{,2..5} (5 alike) : Sum  Inputs=|++
  Throttle : Constant  Value=bias.throttle
  cmds : Outport
  wires:
  Right Roll Spoiler Schedule/1 -> Gain11/1, Gain14/1
  Left Roll Spoiler Schedule/1 -> Gain13/1, Gain12/1
  Gain12/1 -> Bus Creator/11  "SPLLIB"
  Gain13/1 -> Bus Creator/12  "SPLLOB"
  Gain14/1 -> Bus Creator/13  "SPLRIB"
  Gain11/1 -> Bus Creator/14  "SPLROB"
  Gain16/1 -> Bus Creator/15  "FLAPLIB"
  Gain17/1 -> Bus Creator/16  "FLAPLOB"
  Gain18/1 -> Bus Creator/17  "FLAPRIB"
  Gain15/1 -> Bus Creator/18  "FLAPROB"
  Gain23/1 -> Bus Creator/1  "THROTL"
  Gain2/1 -> Bus Creator/2  "THROTR"
  Gain6/1 -> Bus Creator/4  "ELLIB"
  Gain7/1 -> Bus Creator/3  "ELLOB"
  Gain8/1 -> Bus Creator/5  "ELROB"
  Gain22/1 -> Bus Creator/6  "ELRIB"
  Gain1/1 -> Bus Creator/7  "AILL"
  Gain3/1 -> Bus Creator/8  "AILR"
  Gain4/1 -> Bus Creator/9  "RUDU"
  Gain5/1 -> Bus Creator/10  "RUDL"
  Sum3/1 -> Gain7/1, Gain6/1, Gain8/1, Gain22/1
  Aileron/1 -> Sum/2
  Elevator/1 -> Sum3/2
  Sum/1 -> Gain1/1, Gain3/1
  Sum2/1 -> Gain4/1, Gain5/1
  Rudder/1 -> Sum2/2
  Flaps/1 -> Sum4/2
  Constant2/1 -> Sum4/1
  Sum4/1 -> Gain16/1, Gain17/1, Gain18/1, Gain15/1
  Ground1/1 -> Sum/1
  Ground2/1 -> Sum2/1
  Gain19/1 -> Bus Creator/20  "BRAKE"
  Gear/1 -> Gain20/1
  Constant3/1 -> Gain19/1, Gain21/1
  Bus Creator/1 -> cmds/1
  Gain20/1 -> Bus Creator/19  "GEAR"
  Gain21/1 -> Bus Creator/21  "STEER"
  Ground/1 -> Sum3/1
  Constant/1 -> Right Roll Spoiler Schedule/1, Left Roll Spoiler Schedule/1
  Throttle/1 -> Sum5/2
  Constant1/1 -> Sum5/1
  Sum5/1 -> Gain2/1, Gain23/1
  Gear1/1 -> Gain9/1
  Gain9/1 -> Bus Creator/22  "STAB"

== system gtm_design_baseline3/Aircraft Model/Aero/Dynamic Derviatives/Forced Oscillation with Damage Increments/Damage Effects-Increments ==
  alpha : Inport
  pqr : Inport  Port=2
  DamageCase : Inport  Port=3
  CY derivative increment due to rates : simulink_need_slupdate/Interpolation (n-D) using PreLookup  numDimsPopupSelect=3  explicitNumDims=2  table=squeeze(Aero.dC6_damage.ddinc.data(:,:,:,2))  interpMethod=Linear  extrapMethod=Linear  rangeErrorMode=None  NumSelectionDims=2
  Constant : Constant  Value=uint32(1)
  Constant1 : Constant  Value=[0:2]  OutDataTypeStr=uint32
  Data Type Conversion : DataTypeConversion  OutDataTypeStr=uint32  SaturateOnIntegerOverflow=off  RndMeth=Floor
  PreLookup Index Search : simulink_need_slupdate/PreLookup Index Search  bpData=Aero.dC6_damage.ddinc.alpha  searchMode=Binary Search  cacheBpFlag=on  outputFlag=off  IndexDataType=uint32  extrapMode=Linear Extrapolation  rangeErrorMode=None
  Product : Product  RndMeth=Zero
  Subtract : Sum  Inputs=+-
  Sum of Elements : Sum  Inputs=+
  Increment : Outport
  wires:
  Subtract/1 -> CY derivative increment due to rates/2
  Data Type Conversion/1 -> Subtract/1
  Constant/1 -> Subtract/2
  Constant1/1 -> CY derivative increment due to rates/3
  PreLookup Index Search/1 -> CY derivative increment due to rates/1
  DamageCase/1 -> Data Type Conversion/1
  alpha/1 -> PreLookup Index Search/1
  CY derivative increment due to rates/1 -> Product/1
  pqr/1 -> Product/2
  Product/1 -> Sum of Elements/1
  Sum of Elements/1 -> Increment/1

== system gtm_design_baseline3/Aircraft Model/Aero/Dynamic Derviatives/Forced Oscillation with Damage Increments/Damage Effects-Scaling ==
  alpha : Inport
  DamageCase : Inport  Port=2
  Constant : Constant  Value=uint32(1)
  Constant1 : Constant  Value=[0:5]  OutDataTypeStr=uint32
  Constant2 : Constant  Value=[0:5]  OutDataTypeStr=uint32
  Constant3 : Constant  Value=[0:5]  OutDataTypeStr=uint32
  Constant4 : Constant  Value=uint32(1)
  Constant5 : Constant  Value=uint32(1)
  DamageCase3 : InportShadow  Port=2
  DamageCase4 : InportShadow  Port=2
  PreLookup Index Search : simulink_need_slupdate/PreLookup Index Search  bpData=Aero.dC6_damage.ddscale.alpha  searchMode=Binary Search  cacheBpFlag=on  outputFlag=off  IndexDataType=uint32  extrapMode=Linear Extrapolation  rangeErrorMode=None
  Subtract : Sum  Inputs=+-
  Subtract1 : Sum  Inputs=+-
  Subtract2 : Sum  Inputs=+-
  p : simulink_need_slupdate/Interpolation (n-D) using PreLookup  numDimsPopupSelect=3  explicitNumDims=2  table=squeeze(Aero.dC6_damage.ddscale.data(:,:,1,:))  interpMethod=Linear  extrapMethod=None - Clip  rangeErrorMode=None  NumSelectionDims=2
  q : simulink_need_slupdate/Interpolation (n-D) using PreLookup  numDimsPopupSelect=3  explicitNumDims=2  table=squeeze(Aero.dC6_damage.ddscale.data(:,:,2,:))  interpMethod=Linear  extrapMethod=None - Clip  rangeErrorMode=None  NumSelectionDims=2
  r : simulink_need_slupdate/Interpolation (n-D) using PreLookup  numDimsPopupSelect=3  explicitNumDims=2  table=squeeze(Aero.dC6_damage.ddscale.data(:,:,3,:))  interpMethod=Linear  extrapMethod=None - Clip  rangeErrorMode=None  NumSelectionDims=2
  Scaling_r : Outport
  Scaling_q : Outport  Port=2
  Scaling_p : Outport  Port=3
  wires:
  DamageCase4/1 -> Subtract2/1
  Subtract2/1 -> p/2
  DamageCase3/1 -> Subtract1/1
  Subtract1/1 -> q/2
  Constant5/1 -> Subtract2/2
  Constant4/1 -> Subtract1/2
  DamageCase/1 -> Subtract/1
  Subtract/1 -> r/2
  Constant/1 -> Subtract/2
  alpha/1 -> PreLookup Index Search/1
  r/1 -> Scaling_r/1
  PreLookup Index Search/1 -> r/1, q/1, p/1
  q/1 -> Scaling_q/1
  p/1 -> Scaling_p/1
  Constant1/1 -> r/3
  Constant2/1 -> q/3
  Constant3/1 -> p/3

== system gtm_design_baseline3/Aircraft Model/Aero/Dynamic Derviatives/Forced Oscillation with Damage Increments/Forced Oscillation ==
  alpha : Inport
  pqr : Inport  Port=2
  Assignment to Lateral : Assignment  IndexMode=Zero-based  IndexOptions=Index vector (dialog)  Indices=[1 3 5]  OutputSizes=[1 1]
  Assignment to Lateral1 : Assignment  IndexMode=Zero-based  IndexOptions=Index vector (dialog)  Indices=[1 3 5]  OutputSizes=[1 1]
  Assignment to Longitudinal : Assignment  IndexMode=Zero-based  IndexOptions=Index vector (dialog)  Indices=[0 2 4]  OutputSizes=[1 1]
  Constant : Constant  Value=zeros(6,1)
  Constant1 : Constant  Value=[0:2]  OutDataTypeStr=uint32
  Constant2 : Constant  Value=[0:2]  OutDataTypeStr=uint32
  Constant3 : Constant  Value=[0:2]  OutDataTypeStr=uint32
  Constant4 : Constant  Value=zeros(6,1)
  Constant5 : Constant  Value=zeros(6,1)
  Demux : Demux  Outputs=3
  PreLookup Index Search : simulink_need_slupdate/PreLookup Index Search  bpData=Aero.dC3_q.alpha  searchMode=Binary Search  cacheBpFlag=on  outputFlag=off  IndexDataType=uint32  extrapMode=Linear Extrapolation  rangeErrorMode=None
  PreLookup Index Search1 : simulink_need_slupdate/PreLookup Index Search  bpData=Aero.dC3_r.rhat  searchMode=Binary Search  cacheBpFlag=on  outputFlag=off  IndexDataType=uint32  extrapMode=Linear Extrapolation  rangeErrorMode=None
  PreLookup Index Search2 : simulink_need_slupdate/PreLookup Index Search  bpData=Aero.dC3_p.phat  searchMode=Binary Search  cacheBpFlag=on  outputFlag=off  IndexDataType=uint32  extrapMode=Linear Extrapolation  rangeErrorMode=None
  PreLookup Index Search3 : simulink_need_slupdate/PreLookup Index Search  bpData=Aero.dC3_q.qhat  searchMode=Binary Search  cacheBpFlag=on  outputFlag=off  IndexDataType=uint32  extrapMode=Linear Extrapolation  rangeErrorMode=None
  PreLookup Index Search4 : simulink_need_slupdate/PreLookup Index Search  bpData=Aero.dC3_p.alpha  searchMode=Binary Search  cacheBpFlag=on  outputFlag=off  IndexDataType=uint32  extrapMode=Linear Extrapolation  rangeErrorMode=None
  PreLookup Index Search5 : simulink_need_slupdate/PreLookup Index Search  bpData=Aero.dC3_r.alpha  searchMode=Binary Search  cacheBpFlag=on  outputFlag=off  IndexDataType=uint32  extrapMode=Linear Extrapolation  rangeErrorMode=None
  pitch : simulink_need_slupdate/Interpolation (n-D) using PreLookup  numDimsPopupSelect=3  explicitNumDims=2  table=Aero.dC3_q.data  interpMethod=Linear  extrapMethod=None - Clip  rangeErrorMode=None  NumSelectionDims=1
  roll : simulink_need_slupdate/Interpolation (n-D) using PreLookup  numDimsPopupSelect=3  explicitNumDims=2  table=Aero.dC3_p.data  interpMethod=Linear  extrapMethod=None - Clip  rangeErrorMode=None  NumSelectionDims=1
  yaw : simulink_need_slupdate/Interpolation (n-D) using PreLookup  numDimsPopupSelect=3  explicitNumDims=2  table=Aero.dC3_r.data  interpMethod=Linear  extrapMethod=None - Clip  rangeErrorMode=None  NumSelectionDims=1
  dC6_p : Outport
  dC6_q : Outport  Port=2
  dC6_r : Outport  Port=3
  wires:
  alpha/1 -> PreLookup Index Search4/1, PreLookup Index Search5/1, PreLookup Index Search/1
  pqr/1 -> Demux/1
  Constant1/1 -> pitch/3
  Demux/2 -> PreLookup Index Search3/1
  Demux/1 -> PreLookup Index Search2/1
  Demux/3 -> PreLookup Index Search1/1
  Constant2/1 -> roll/3
  Constant3/1 -> yaw/3
  Constant/1 -> Assignment to Longitudinal/1
  pitch/1 -> Assignment to Longitudinal/2
  roll/1 -> Assignment to Lateral/2
  Constant4/1 -> Assignment to Lateral/1
  Constant5/1 -> Assignment to Lateral1/1
  yaw/1 -> Assignment to Lateral1/2
  PreLookup Index Search1/1 -> yaw/2
  PreLookup Index Search2/1 -> roll/2
  PreLookup Index Search3/1 -> pitch/2
  Assignment to Lateral/1 -> dC6_p/1
  Assignment to Lateral1/1 -> dC6_r/1
  Assignment to Longitudinal/1 -> dC6_q/1
  PreLookup Index Search/1 -> pitch/1
  PreLookup Index Search4/1 -> roll/1
  PreLookup Index Search5/1 -> yaw/1

== system gtm_design_baseline3/Aircraft Model/Aero/Dynamic Derviatives/Forced Oscillation with Damage Increments/Normalize ==
  pqr : Inport
  TAS : Inport  Port=2
  AC_Params : Inport  Port=3
  Bus Selector2 : BusSelector  OutputSignals=B,Cbar,B
  Gain : Gain  Gain=2*(1.689)
  Mux : Mux  Inputs=3
  Product3 : Product  Inputs=**/  RndMeth=Zero
  Saturation1 : Saturate  UpperLimit=10000  LowerLimit=1
  pqrhat : Outport
  wires:
  Mux/1 -> Product3/2
  Bus Selector2/3 -> Mux/3  "<B>"
  Bus Selector2/2 -> Mux/2  "<Cbar>"
  Bus Selector2/1 -> Mux/1  "<B>"
  Product3/1 -> pqrhat/1
  Gain/1 -> Product3/3
  pqr/1 -> Product3/1
  Saturation1/1 -> Gain/1
  AC_Params/1 -> Bus Selector2/1
  TAS/1 -> Saturation1/1
